simulink model "VehiclePlant"  (R2024a)
settings: configuration reference "standardSILConfiguraitonParams" (kept outside this file)
values from neighbouring files (symbols this model uses):
  vehicleParams = evalin('base', 'vehicleParams')    [testVehicleSIL.m]
settings Model: Creator=GTAR  LastModifiedBy=jerem
settings ConfigSetRef: SourceName=standardSILConfiguraitonParams  SourceLocation=Base Workspace

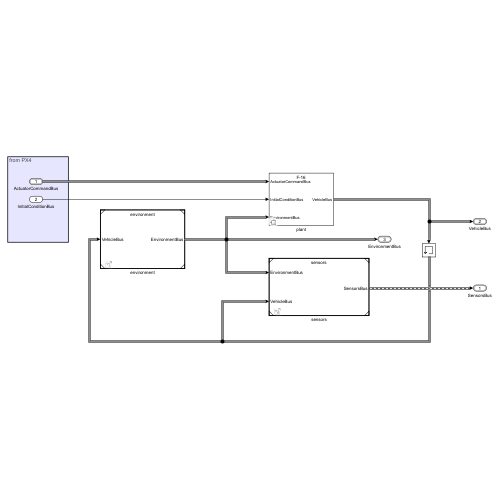
[thumbnail: Simulink's stored preview of the top-level diagram]
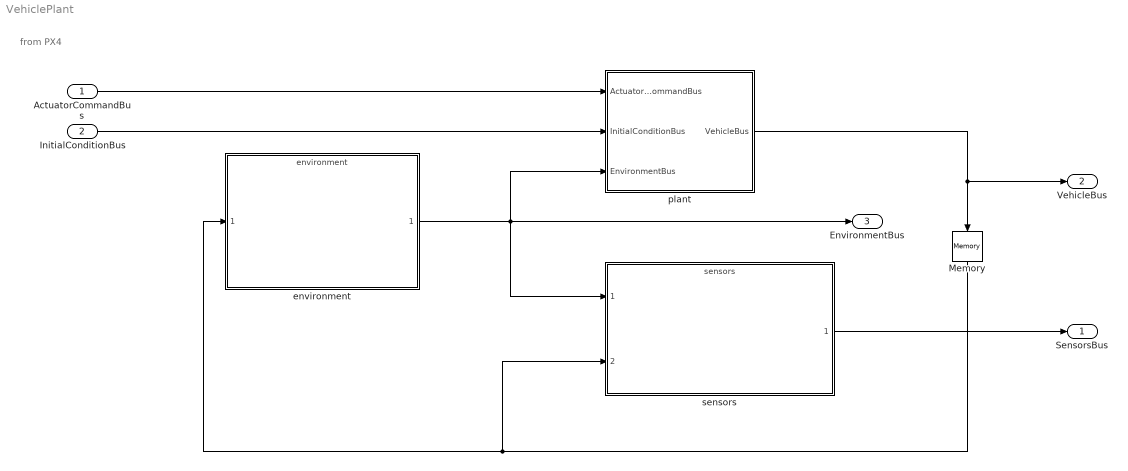
== system VehiclePlant ==
  note: from PX4
  ActuatorCommandBus : Inport  OutDataTypeStr=Bus: ActuatorCommandBus  LockScale=on
  InitialConditionBus : Inport  Port=2
  Memory : Memory
  environment : ModelReference  ModelNameDialog=environment.slx  SimulationMode=Normal  ModelReferenceVersion=1.13
  plant : Subsystem  Variant=on
  sensors : ModelReference  ModelNameDialog=sensors.slx  SimulationMode=Normal  ModelReferenceVersion=1.26
  SensorsBus : Outport  OutDataTypeStr=Bus: SensorsBus
  VehicleBus : Outport  Port=2  OutDataTypeStr=Bus: VehicleBus
  EnvironmentBus : Outport  Port=3  OutDataTypeStr=Bus: EnvironmentBus
  wires:
  sensors/1 -> SensorsBus/1
  ActuatorCommandBus/1 -> plant/1(ActuatorCommandBus)
  environment/1 -> sensors/1, EnvironmentBus/1, plant/3(EnvironmentBus)
  InitialConditionBus/1 -> plant/2(InitialConditionBus)
  Memory/1 -> sensors/2, environment/1
  plant/1(VehicleBus) -> VehicleBus/1, Memory/1

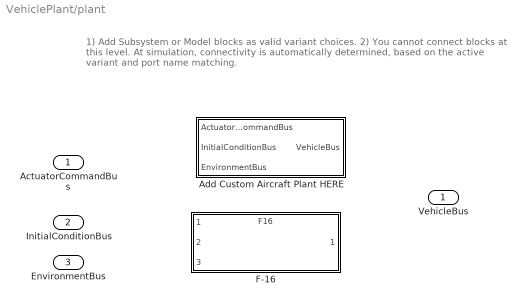
== system VehiclePlant/plant ==
  note: 1) Add Subsystem or Model blocks as valid variant choices.
      | 2) You cannot connect blocks at this level. At simulation, connectivity is automatically
      | determined, based on the active variant and port name matching.
  ActuatorCommandBus : Inport  OutDataTypeStr=Bus: ActuatorCommandBus  LockScale=on
  InitialConditionBus : Inport  Port=2
  EnvironmentBus : Inport  Port=3  OutDataTypeStr=Bus: EnvironmentBus
  Add Custom Aircraft Plant HERE : Subsystem  VariantControl="strcmp(vehicleParams.type ,\"Custom\")"
  F-16 : ModelReference  ModelNameDialog=F16.slx  VariantControl="strcmp(vehicleParams.type ,\"F-16\")"  ModelReferenceVersion=1.87
  VehicleBus : Outport

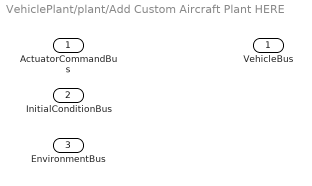
== system VehiclePlant/plant/Add Custom Aircraft Plant HERE ==
  ActuatorCommandBus : Inport
  InitialConditionBus : Inport  Port=2
  EnvironmentBus : Inport  Port=3
  VehicleBus : Outport
